simulink model "temperature_network"  (R2024b)
settings: Solver=VariableStepAuto  StartTime=0.0  StopTime=60  RelTol=1e-3
values from neighbouring files (symbols this model uses):
  Ptest_Thermal_Network = 50    [init_pv_inverter.m]
  Ta = test_cases(k,2)    [blindval.m]    (also in init_pv_inverter.m = 25)
libraries: fl_lib x5, nesl_utility x3, ee_lib x1
settings Model: Creator=tf  LastModifiedBy=tf

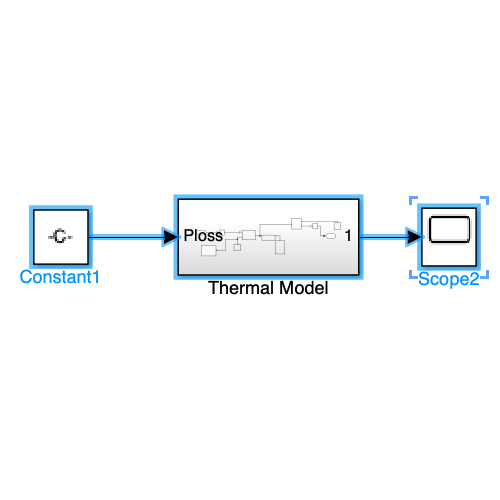
[thumbnail: Simulink's stored preview of the top-level diagram]
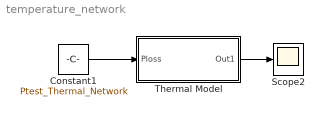
== system temperature_network ==
  Constant1 : Constant  Value=Ptest_Thermal_Network
  Scope2 : Scope
  Thermal Model : Subsystem
  wires:
  Constant1/1 -> Thermal Model/1(Ploss)
  Thermal Model/1(Out1) -> Scope2/1

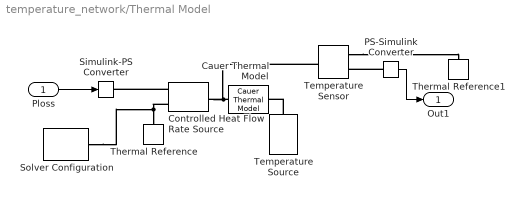
== system temperature_network/Thermal Model ==
  Ploss : Inport
  Cauer Thermal Model : ee_lib/Passive/Thermal/Cauer Thermal Model  parameterize_foster=false  resistance_data=Rth K/W  tau_data=tau_th s  resistance_data_foster=[.0016, .0043, .0013, .0014] K/W  tau_data_foster=[.0068, .064, .32, 2] s  Tvec_specify=on  Tvec_priority=None  Tvec=Tinit K  Tvec_nominal_specify=off  Tvec_nominal_value=1  Tvec_nominal_unit=K  Q_A_specify=off  Q_A_priority=None  Q_A=0 W  Q_A_nominal_specify=off  Q_A_nominal_value=1  Q_A_nominal_unit=W  Q_B_specify=off  Q_B_priority=None  Q_B=0 W  Q_B_nominal_specify=off  Q_B_nominal_value=1  Q_B_nominal_unit=W
      settings: InternalSimscapePortConfiguration="{\"Bottom\":[],\"Left\":[{\"id\":\"A\",\"label\":\"A\",\"type\":\"foundation.thermal.thermal\"}],\"Right\":[{\"id\":\"B\",\"label\":\"B\",\"type\":\"foundation.thermal.thermal\"}],\"Top\":[]}"
  Controlled Heat Flow Rate Source : fl_lib/Thermal/Thermal Sources/Controlled Heat Flow Rate Source
  PS-Simulink Converter : nesl_utility/PS-Simulink Converter  PhysicalDomain=network_engine_domain  SubClassName=ps_output  LeftPortType=input  RightPortType=output  PseudoPeriodic=off  Frequencies=[]  VectorFormat=inherit  Unit=inherit  AffineConversion=off
  Simulink-PS Converter : nesl_utility/Simulink-PS Converter  PhysicalDomain=network_engine_domain  SubClassName=ps_input  LeftPortType=input  RightPortType=output  PseudoPeriodic=off  Frequencies=[]  NoiseDistribution=none  NoiseParameters=[]  Unit=W  AffineConversion=off  FilteringAndDerivatives=provide  SimscapeFilterOrder=1  InputFilterTimeConstant=0.001  UdotUserProvided=0
  Solver Configuration : nesl_utility/Solver Configuration  PhysicalDomain=network_engine_domain  SubClassName=solver  LeftPortType=input  RightPortType=generic  Tones=[]  Harmonics=[]  SimulateNoise=off  Profile=off  UseLocalSampling=off  EnableSwitchedLinearOptims=on  FrequencyDomain=off  UseCCode=off  RelTol=0.001  AbsTol=0.001  MinStep=1e-09  ToWorkspace=off  RevertToSquareIcSolve=off  NumHomotopyIterations=100  PhasorMode=off  PhasorModeNumHarmonics=1  ConsistencySolver=NEWTON_XTOL_AFTER_FTOL  IndexReductionMethod=DerivativeReplacement  DoDC=off  ResidualTolerance=1e-09  ConsistencyTolSource=GLOBAL  ConsistencyAbsTol=0.001  ConsistencyRelTol=0.001  ConsistencyTolFactor=0.001  UseLocalSolver=off  LocalSolverChoice=NE_BACKWARD_EULER_ADVANCER  ResolveIndetEquations=on  FunctionEvalNumThread=1  LocalSolverSampleTime=0.001  DoFixedCost=off  MaxNonlinIter=3  MaxModeIter=2  ComputeImpulses=off  ImpulseIterations=2  LinearAlgebra=auto  LinearAlgebraNumThread=0  EquationFormulation=NE_TIME_EF  DelaysMemoryBudget=1024  AutomaticFiltering=on  FilteringTimeConstant=0.001  PartitionStorageMethod=AS_NEEDED  PartitionMemoryBudget=1024  PartitionMethod=ROBUST  MultibodyUseLocalSolver=off  MultibodyLocalSolverChoice=ODE1  MultibodyLocalSolverSampleTime=0.001
  Temperature Sensor : fl_lib/Thermal/Thermal Sensors/Temperature Sensor  temperature_measure=foundation.enum.MeasurementReference.difference
  Temperature Source : fl_lib/Thermal/Thermal Sources/Temperature Source  temperature=Ta + 273.15 K
  Thermal Reference : fl_lib/Thermal/Thermal Elements/Thermal Reference
  Thermal Reference1 : fl_lib/Thermal/Thermal Elements/Thermal Reference
  Out1 : Outport
  wires:
  Ploss/1 -> Simulink-PS Converter/1
  PS-Simulink Converter/1 -> Out1/1
  connections:
  Controlled Heat Flow Rate Source/RConn1 -- Simulink-PS Converter/RConn1
  Controlled Heat Flow Rate Source/LConn1 -- Cauer Thermal Model/LConn1 -- Temperature Sensor/LConn1
  Temperature Source/LConn1 -- Cauer Thermal Model/RConn1
  Thermal Reference/LConn1 -- Controlled Heat Flow Rate Source/RConn2 -- Solver Configuration/RConn1
  PS-Simulink Converter/LConn1 -- Temperature Sensor/RConn2
  Temperature Sensor/RConn1 -- Thermal Reference1/LConn1
